simulink model "MLP_ROM_MOS"  (R2025a)
settings: Solver=FixedStepAuto  StartTime=0.0  StopTime=5000  RelTol=1e-3
undefined symbols (not defined in the file or in its folder): b5579956, trainingOutputMLP
libraries: deeplib x1
settings Model: SILPILSystemUnderTest=refmodels  SILPILSimulationModeTopModel=accelerator  Creator=skeshavm
settings OptimizationCC: DefaultParameterBehavior=Inlined  UseDivisionForNetSlopeComputation=on  GainParamInheritBuiltInType=on  UseFloatMulNetSlope=on  InheritOutputTypeSmallerThanSingle=on  DefaultUnderspecifiedDataType=single  EnhancedBackFolding=on  PassReuseOutputArgsAs=Individual arguments  ZeroExternalMemoryAtStartup=off  ZeroInternalMemoryAtStartup=off  MaxStackSize=200000  OptimizeBlockOrder=speed  DifferentSizesBufferReuse=on  UseRowMajorAlgorithm=on  OptimizationCustomize=off  EfficientTunableParamExpr=on
settings DebuggingCC: ParameterTunabilityLossMsg=error
settings SFSimCC: MATLABDynamicMemAlloc=off
settings RTWCC: SystemTargetFile=ert.tlc  GenCodeOnly=on  TemplateMakefile=ert_default_tmf  CodeExecutionProfiling=on  TargetLang=C++  Description=Embedded Coder
settings CodeAppCC: ForceParamTrailComments=on  IgnoreCustomStorageClasses=off  OperatorAnnotations=on  SimulinkDataObjDesc=on  SFDataObjDesc=on  InsertBlockDesc=on
settings ERTTargetCC: ExtModeTransport=0.0  ExtModeStaticAlloc=off  ExtModeMexFile=ext_comm  ExtModeIntrfLevel=Level1  RootIOFormat=Structure reference  ERTCustomFileTemplate=example_file_process.tlc  CodeInterfacePackaging=C++ class

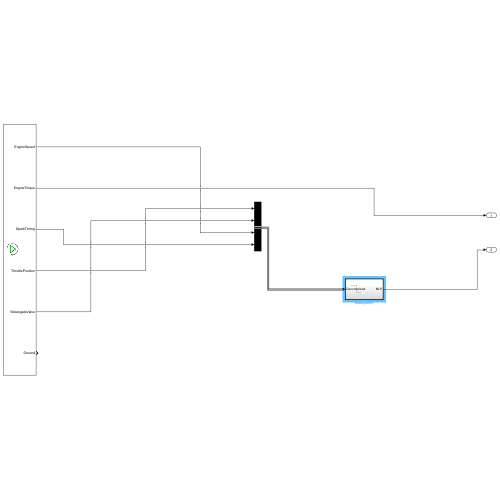
[thumbnail: Simulink's stored preview of the top-level diagram]
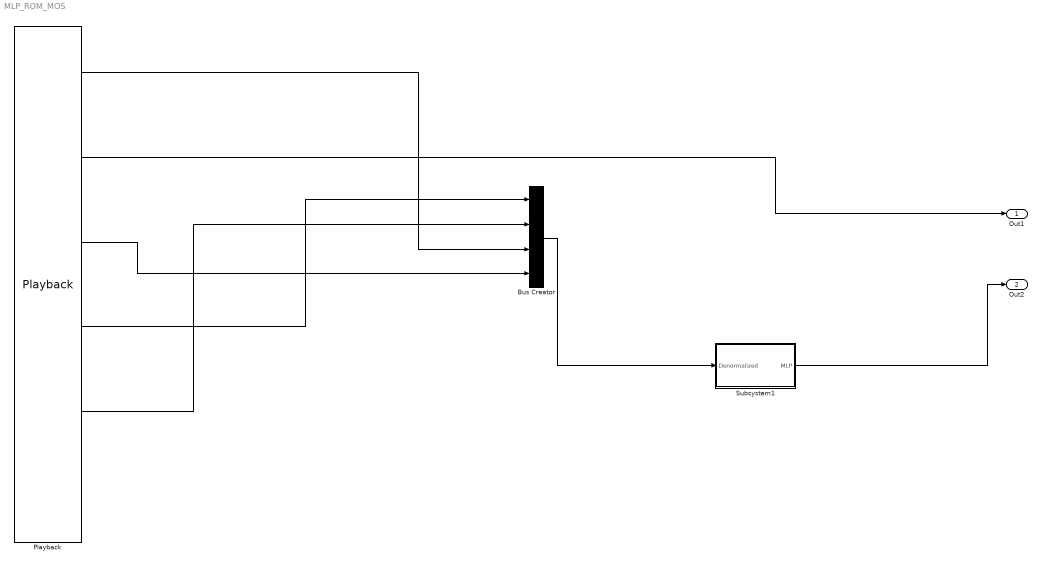
== system MLP_ROM_MOS ==
  Bus Creator : BusCreator  Inputs=4
  Playback : Playback  NumPorts=6  PartName=b5579956-5d05-46cb-96b4-8c90d5937c62  TablePosition=Bottom
  Subsystem1 : Subsystem  TreatAsAtomicUnit=on
  Out1 : Outport
  Out2 : Outport  Port=2
  wires:
  Playback/2 -> Out1/1
  Playback/4 -> Bus Creator/1
  Playback/5 -> Bus Creator/2
  Playback/1 -> Bus Creator/3
  Playback/3 -> Bus Creator/4
  Bus Creator/1 -> Subsystem1/1(Denormalized)
  Subsystem1/1(MLP) -> Out2/1

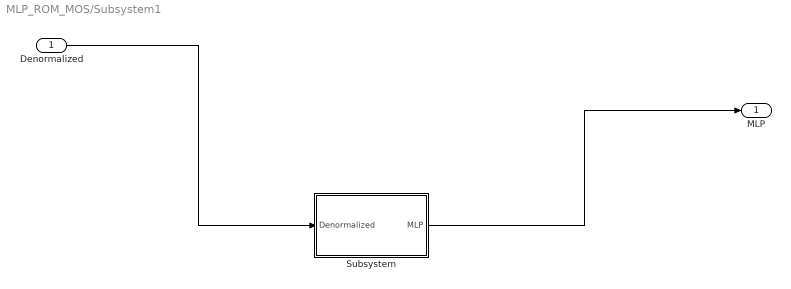
== system MLP_ROM_MOS/Subsystem1 ==
  Denormalized : Inport
  Subsystem : Subsystem
  MLP : Outport
  wires:
  Subsystem/1(MLP) -> MLP/1
  Denormalized/1 -> Subsystem/1(Denormalized)

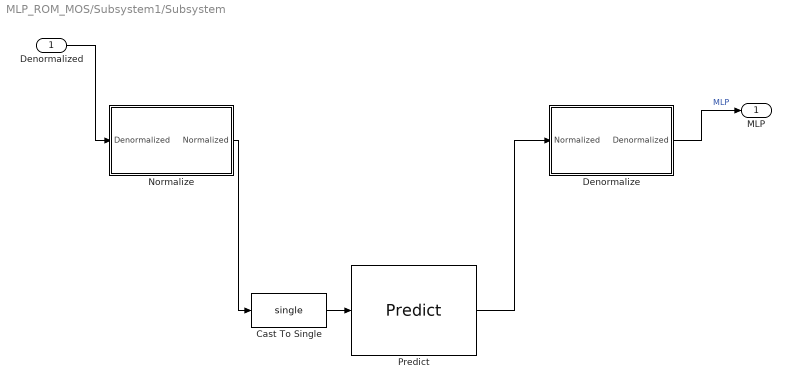
== system MLP_ROM_MOS/Subsystem1/Subsystem ==
  Denormalized : Inport
  Cast To Single : DataTypeConversion  OutDataTypeStr=single  SaturateOnIntegerOverflow=off  RndMeth=Floor
  Denormalize : Subsystem
  Normalize : Subsystem
  Predict : deeplib/Predict  Network=Network from MAT-file  NetworkFunction=squeezenet  NetworkFilePath=SIMLP.mat  MiniBatchSize=128  InputDataFormats={ 'ThrottlePosition, WastegateValve, EngineSpeed, SparkTiming', 'CB' }  Predictions=on  Activations={}  ForceInterpretedSim=off  EnableDLNetwork=on  LastKnownNetworkFilePath='SIMLP.mat'  LastKnownNetworkTimeStamp=739875.919363425928167998790740966796875
  MLP : Outport
  wires:
  Predict/1 -> Denormalize/1(Normalized)
  Cast To Single/1 -> Predict/1
  Normalize/1(Normalized) -> Cast To Single/1
  Denormalized/1 -> Normalize/1(Denormalized)
  Denormalize/1(Denormalized) -> MLP/1  "MLP"

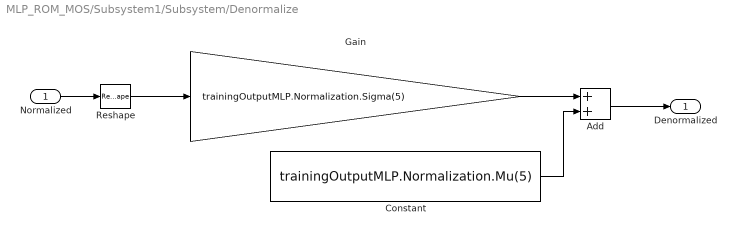
== system MLP_ROM_MOS/Subsystem1/Subsystem/Denormalize ==
  Normalized : Inport
  Add : Sum
  Constant : Constant  Value=trainingOutputMLP.Normalization.Mu(5)
  Gain : Gain  Gain=trainingOutputMLP.Normalization.Sigma(5)  OutDataTypeStr=single
  Reshape : Reshape
  Denormalized : Outport
  wires:
  Constant/1 -> Add/2
  Gain/1 -> Add/1
  Add/1 -> Denormalized/1
  Normalized/1 -> Reshape/1
  Reshape/1 -> Gain/1

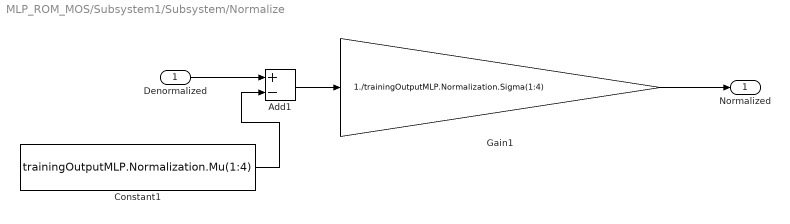
== system MLP_ROM_MOS/Subsystem1/Subsystem/Normalize ==
  Denormalized : Inport
  Add1 : Sum  Inputs=+-
  Constant1 : Constant  Value=trainingOutputMLP.Normalization.Mu(1:4)
  Gain1 : Gain  Gain=1./trainingOutputMLP.Normalization.Sigma(1:4)
  Normalized : Outport
  wires:
  Add1/1 -> Gain1/1
  Constant1/1 -> Add1/2
  Gain1/1 -> Normalized/1
  Denormalized/1 -> Add1/1
